simulink model "chap7_4sim"  (Simulink 5.0)
settings: Solver=ode45  StartTime=0.0  StopTime=10  FixedStep=0.001  RelTol=1e-3
settings Model: LastModifiedBy=Administrator  ExtModeTrigMode=oneshot  ExtModeArmWhenConnect=off  LimitDataPoints=off  BooleanDataType=off

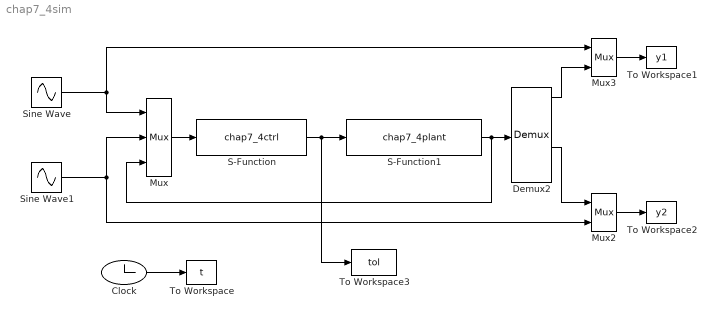
== system chap7_4sim ==
  Clock : Clock
  Demux2 : Demux
  Mux : Mux  Inputs=3
  Mux2 : Mux  Inputs=2
  Mux3 : Mux  Inputs=2
  S-Function : S-Function  FunctionName=chap7_4ctrl
  S-Function1 : S-Function  FunctionName=chap7_4plant
  Sine Wave : Sin  Frequency=pi  Phase=pi/2  SampleTime=0
  Sine Wave1 : Sin  Frequency=pi  SampleTime=0
  To Workspace : ToWorkspace  VariableName=t  SampleTime=-1  SaveFormat=Array
  To Workspace1 : ToWorkspace  VariableName=y1  SampleTime=-1  SaveFormat=Array
  To Workspace2 : ToWorkspace  VariableName=y2  SampleTime=-1  SaveFormat=Array
  To Workspace3 : ToWorkspace  VariableName=tol  SampleTime=-1  SaveFormat=Array
  wires:
  Mux/1 -> S-Function/1
  Mux2/1 -> To Workspace2/1
  Sine Wave/1 -> Mux/1, Mux3/1
  Mux3/1 -> To Workspace1/1
  S-Function/1 -> S-Function1/1, To Workspace3/1
  Sine Wave1/1 -> Mux/2, Mux2/2
  Demux2/1 -> Mux3/2
  S-Function1/1 -> Demux2/1, Mux/3
  Demux2/3 -> Mux2/1
  Clock/1 -> To Workspace/1
